simulink model "control_remolque"  (R2020a)
settings: Solver=VariableStepAuto  StartTime=0.0  StopTime=5  RelTol=1e-3
settings Model: Creator=leo_g  LastModifiedBy=leo_g

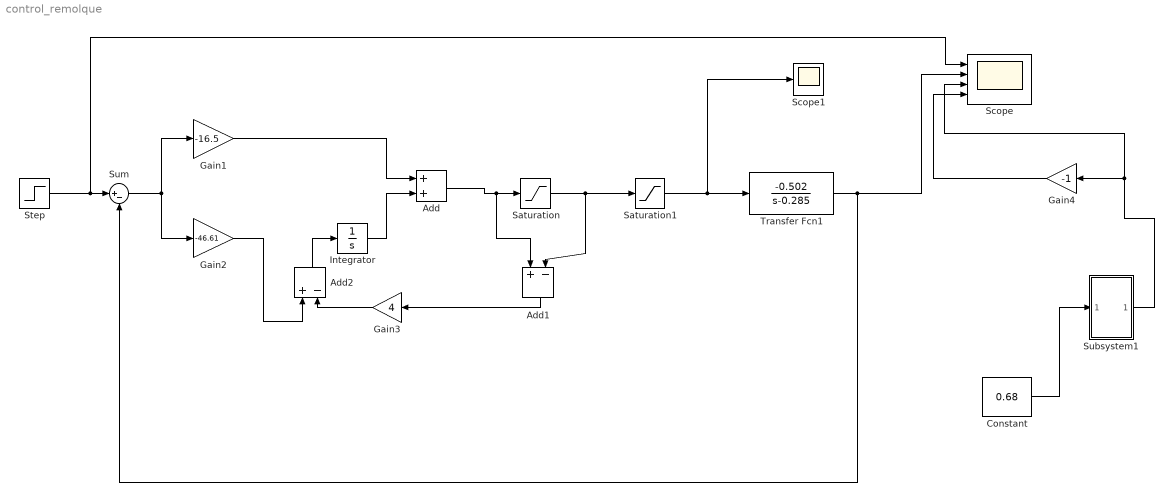
== system control_remolque ==
  Add : Sum
  Add1 : Sum  Inputs=+-
  Add2 : Sum  Inputs=+-
  Constant : Constant  Value=0.68
  Gain1 : Gain  Gain=-16.5
  Gain2 : Gain  Gain=-46.61
  Gain3 : Gain  Gain=4
  Gain4 : Gain  Gain=-1
  Integrator : Integrator
  Saturation : Saturate  UpperLimit=0.6  LowerLimit=-0.6
  Saturation1 : Saturate  UpperLimit=0.6  LowerLimit=-0.6
  Scope : Scope  NumInputPorts=4
  Scope1 : Scope
  Step : Step  Time=0  After=0.7853  SampleTime=0
  Subsystem1 : Subsystem
  Sum : Sum  Inputs=|+-
  Transfer Fcn1 : TransferFcn  Numerator=[-0.502]  Denominator=[1 -0.285]
  wires:
  Transfer Fcn1/1 -> Scope/2, Sum/2
  Step/1 -> Sum/1, Scope/1
  Add1/1 -> Gain3/1
  Constant/1 -> Subsystem1/1(In1)
  Gain1/1 -> Add/1
  Integrator/1 -> Add/2
  Saturation/1 -> Saturation1/1, Add1/2
  Gain3/1 -> Add2/2
  Gain2/1 -> Add2/1
  Add2/1 -> Integrator/1
  Add/1 -> Add1/1, Saturation/1
  Subsystem1/1(Out1) -> Scope/3, Gain4/1
  Saturation1/1 -> Transfer Fcn1/1, Scope1/1
  Sum/1 -> Gain2/1, Gain1/1
  Gain4/1 -> Scope/4

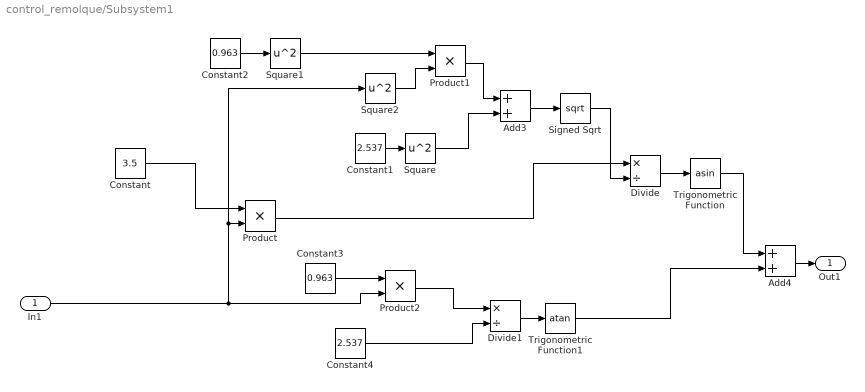
== system control_remolque/Subsystem1 ==
  In1 : Inport
  Add3 : Sum
  Add4 : Sum
  Constant : Constant  Value=3.5
  Constant1 : Constant  Value=2.537
  Constant2 : Constant  Value=0.963
  Constant3 : Constant  Value=0.963
  Constant4 : Constant  Value=2.537
  Divide : Product  Inputs=*/
  Divide1 : Product  Inputs=*/
  Product : Product
  Product1 : Product
  Product2 : Product
  Signed Sqrt : Sqrt  SaturateOnIntegerOverflow=on
  Square : Math  Operator=square  SaturateOnIntegerOverflow=on
  Square1 : Math  Operator=square  SaturateOnIntegerOverflow=on
  Square2 : Math  Operator=square  SaturateOnIntegerOverflow=on
  Trigonometric Function : Trigonometry  Operator=asin
  Trigonometric Function1 : Trigonometry  Operator=atan
  Out1 : Outport
  wires:
  Constant3/1 -> Product2/1
  Product1/1 -> Add3/1
  Square/1 -> Add3/2
  Square2/1 -> Product1/2
  In1/1 -> Product2/2, Square2/1, Product/2
  Add3/1 -> Signed Sqrt/1
  Product/1 -> Divide/1
  Constant2/1 -> Square1/1
  Constant/1 -> Product/1
  Product2/1 -> Divide1/1
  Divide1/1 -> Trigonometric Function1/1
  Square1/1 -> Product1/1
  Trigonometric Function/1 -> Add4/1
  Trigonometric Function1/1 -> Add4/2
  Constant1/1 -> Square/1
  Signed Sqrt/1 -> Divide/2
  Constant4/1 -> Divide1/2
  Divide/1 -> Trigonometric Function/1
  Add4/1 -> Out1/1
